simulink model "sim_cutin"  (Simulink 8.8)
settings: Solver=ode8  StartTime=0.0  StopTime=20  RelTol=1e-3  EnableMultiTasking=on
settings Model: SuppressorTable=22 serialization::archive 11 0 3 0 0 0 0 0  Creator=petter  LastModifiedBy=petter
settings DataIOCC: SaveOutput=off  SaveTime=off
settings DebuggingCC: SolverPrmCheckMsg=warning  MultiTaskDSMMsg=warning  MultiTaskCondExecSysMsg=none  FcnCallInpInsideContextMsg=error
settings GRTTargetCC: CombineOutputUpdateFcns=on  GRTInterface=off

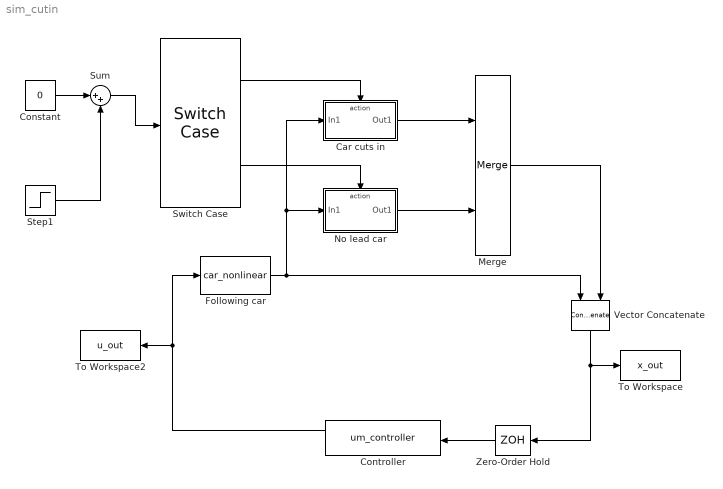
== system sim_cutin ==
  "Car cuts in " : Subsystem  TreatAsAtomicUnit=on
  Constant : Constant  Value=0
  Controller : M-S-Function  FunctionName=um_controller
  Following car : M-S-Function  FunctionName=car_nonlinear  Parameters=25
  Merge : Merge
  No lead car : Subsystem  TreatAsAtomicUnit=on
  Step1 : Step  Time=5  SampleTime=0
  Sum : Sum  Inputs=|++
  Switch Case : SwitchCase
  To Workspace : ToWorkspace  VariableName=x_out  SaveFormat=Structure With Time  SampleTime=-1
  To Workspace2 : ToWorkspace  VariableName=u_out  SaveFormat=Structure With Time  SampleTime=-1
  Vector Concatenate : Concatenate
  Zero-Order Hold : ZeroOrderHold  SampleTime=0.02
  wires:
  Controller/1 -> Following car/1, To Workspace2/1
  Zero-Order Hold/1 -> Controller/1
  No lead car/1(Out1) -> Merge/2
  Merge/1 -> Vector Concatenate/2
  Vector Concatenate/1 -> To Workspace/1, Zero-Order Hold/1
  Constant/1 -> Sum/1
  "Car cuts in "/1(Out1) -> Merge/1
  Switch Case/1 -> "Car cuts in "/Action
  Following car/1 -> "Car cuts in "/1(In1), No lead car/1(In1), Vector Concatenate/1
  Sum/1 -> Switch Case/1
  Step1/1 -> Sum/2
  Switch Case/2 -> No lead car/Action

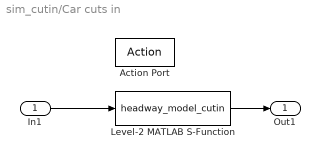
== system sim_cutin/Car cuts in  ==
  In1 : Inport
  Action Port : ActionPort  InitializeStates=reset  ActionType=case
  Level-2 MATLAB S-Function : M-S-Function  FunctionName=headway_model_cutin  Parameters=60,20,3
  Out1 : Outport
  wires:
  In1/1 -> Level-2 MATLAB S-Function/1
  Level-2 MATLAB S-Function/1 -> Out1/1

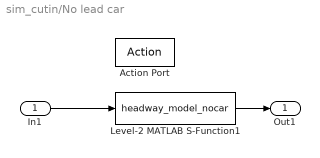
== system sim_cutin/No lead car ==
  In1 : Inport
  Action Port : ActionPort  InitializeStates=reset  ActionType=default
  Level-2 MATLAB S-Function1 : M-S-Function  FunctionName=headway_model_nocar  Parameters=200.1
  Out1 : Outport
  wires:
  In1/1 -> Level-2 MATLAB S-Function1/1
  Level-2 MATLAB S-Function1/1 -> Out1/1
